simulink model "test_feng_ct_packetise"  (Simulink 7.2)
settings: Solver=ode45  StartTime=0.0  StopTime=66000  RelTol=1e-3
libraries: xbsIndex_r4 x152, xps_library x3, casper_library x3
(part 1 of 2)
settings Model: Creator=root  LastModifiedBy=root

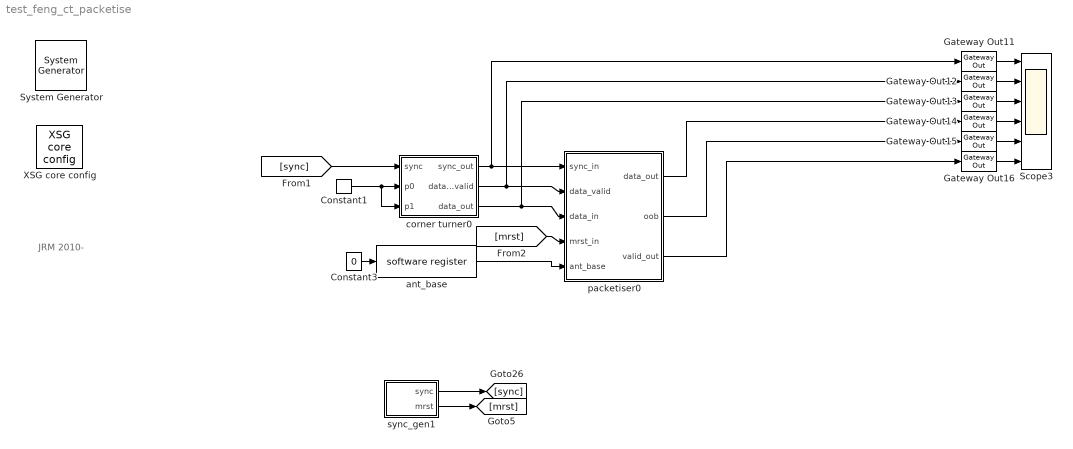
== system test_feng_ct_packetise ==
  note: JRM
      | 2010-
  " System Generator" : xbsIndex_r4/ System Generator  Tag=genX  SystemSampleTime=-1  xilinxfamily=virtex5  part=xc5vsx95t  speed=-1  package=ff1136  synthesis_tool=XST  clock_wrapper=Clock Enables  directory=./r_128w_512_11_r354/sysgen  testbench=off  simulink_period=1  sysclk_period=5  dcm_input_clock_period=100  incr_netlist=off  trim_vbits=Everywhere in SubSystem  dbl_ovrd=According to Block Masks  core_generation=According to Block Masks  run_coregen=off  deprecated_control=off  eval_field=0  block_type=sysgen
      settings: block_version=10.1.3
  Constant1 : xbsIndex_r4/Constant  arith_type=Unsigned  const=0  n_bits=16  bin_pt=0  explicit_period=off  period=1  equ=P=C  opselect=C  inp2=PCIN>>17  opr=+  inp1=P  carry=CIN  dbl_ovrd=off  block_type=constant
  Constant3 : Constant  Value=0  OutDataType=sfix(16)  OutScaling=2^0
  Gateway Out{11..16} (6 alike) : xbsIndex_r4/Gateway Out  hdl_port=off  timing_constraint=None  locs_specified=off  LOCs={}  block_type=gatewayout
      settings: infoedit="Gateway out block.  Converts Xilinx fixed point inputs into ouputs of type Simulink integer, double, or fixed point.<P><P>Hardware notes:  In hardware these blocks become top level output ports or are discarded, depending on how they are configured."  block_version=10.1.3
  Scope3 : Scope  NumInputPorts=6
      settings: YMin=-1~-1~-1~-1~-1~-1  YMax=1~1~1~1~1~1
  XSG core config : xps_library/XSG core config  Tag=xps:xsg  SystemSampleTime=-1  hw_sys=ROACH:sx95t  ibob_linux=off  clk_src=adc0_clk  iBOB_clk_src=sys_clk  BEE2_ctrl_clk_src=sys_clk  BEE2_usr_clk_src=sys_clk  ROACH_clk_src=adc0_clk  CORR_clk_src=sys_clk  gpio_clk_io_group=iBOB:sma  gpio_clk_bit_index=0  clk_rate=800/4  sample_period=1  synthesis_tool=XST  mpc_type=powerpc440_ext
  ant_base : xps_library/software register  Tag=xps:sw_reg  SystemSampleTime=-1  io_dir=From Processor  arith_type=Unsigned  bitwidth=32  bin_pt=0  sample_period=1  gw_name=test_feng_ct_packetise_ant_base_user_data_out
  corner turner0 : Subsystem  mask{num_channels_bits=6, num_spectra_bits=7, which_qdr=qdr0}
      mask prompts: num_channels_bits "Number of freq channels (total 2^?):"; num_spectra_bits "Number of spectra per XAUI packet (2^?):"; which_qdr "QDR to use:"
      mask init:
      | set_param([gcb, '/qdr_ct'], 'which_qdr', which_qdr);
      mask StyleString: edit,edit,popup(qdr0|qdr1)
  packetiser0 : Subsystem  mask{num_spectra_bits=7, ant_bits=1, ant=0}
      mask prompts: num_spectra_bits "Payload length in 64bit words (2^n):"; ant_bits "Number of dual-pol antennas per board (2^n)"; ant "This is antenna number"
      mask help: Package 32 bit data into 64 bits and identify data as coming from antenna 0 or 1
  sync_gen1 : Subsystem
  wires:
  corner turner0/3(data_out) -> Gateway Out13/1, packetiser0/3(data_in)
  corner turner0/2(data_valid) -> Gateway Out12/1, packetiser0/2(data_valid)
  Constant3/1 -> ant_base/1
  ant_base/1 -> packetiser0/5(ant_base)
  Constant1/1 -> corner turner0/3(p1), corner turner0/2(p0)
  [sync] -> corner turner0/1(sync)
  Gateway Out11/1 -> Scope3/1
  Gateway Out12/1 -> Scope3/2
  Gateway Out13/1 -> Scope3/3
  Gateway Out14/1 -> Scope3/4
  Gateway Out15/1 -> Scope3/5
  Gateway Out16/1 -> Scope3/6
  packetiser0/1(data_out) -> Gateway Out14/1
  packetiser0/2(oob) -> Gateway Out15/1
  packetiser0/3(valid_out) -> Gateway Out16/1
  corner turner0/1(sync_out) -> Gateway Out11/1, packetiser0/1(sync_in)
  [mrst] -> packetiser0/4(mrst_in)
  sync_gen1/2(mrst) -> [mrst]
  sync_gen1/1(sync) -> [sync]

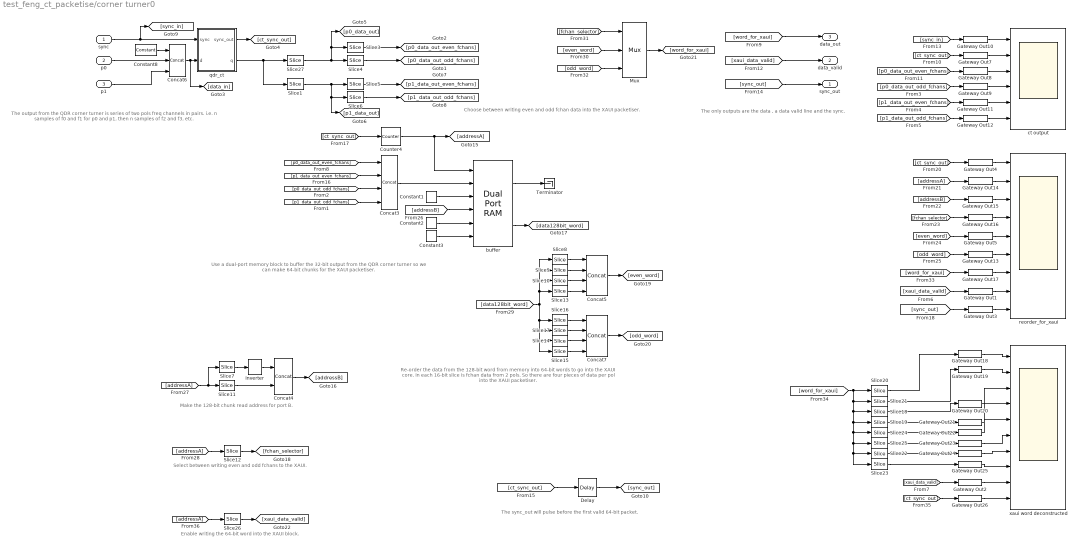
== system test_feng_ct_packetise/corner turner0 ==
  note: Make the 128-bit chunk read address for port B.
  note: Select between writing even and odd fchans to the XAUI.
  note: Re-order the data from the 128-bit word from memory
      | into 64-bit words to go into the XAUI core.
      | In each 16-bit slice is fchan data from 2 pols. So there
      | are four pieces of data per pol into the XAUI packetiser.
  note: Enable writing the 64-bit word into the XAUI block.
  note: The output from the QDR corner turner is series of two pols freq channels in pairs.
      | i.e. n samples of f0 and f1 for p0 and p1, then n samples of f2 and f3, etc.
  note: Use a dual-port memory block to buffer the 32-bit output from the
      | QDR corner turner so we can make 64-bit chunks for the XAUI packetiser.
  note: Choose between writing even and odd fchan data into
      | the XAUI packetiser.
  note: The only outputs are the data , a data valid line and the sync.
  note: The sync_out will pulse before the first valid 64-bit packet.
  sync : Inport  OutDataType=sfix(16)  OutScaling=2^0
  p0 : Inport  Port=2  OutDataType=sfix(16)  OutScaling=2^0
  p1 : Inport  Port=3  OutDataType=sfix(16)  OutScaling=2^0
  Concat3 : xbsIndex_r4/Concat  num_inputs=4  dbl_ovrd=off  block_type=concat
      settings: block_version=10.1.3
  Concat4 : xbsIndex_r4/Concat  num_inputs=2  dbl_ovrd=off  block_type=concat
      settings: block_version=10.1.3
  Concat5 : xbsIndex_r4/Concat  num_inputs=4  dbl_ovrd=off  block_type=concat
      settings: block_version=10.1.3
  Concat6 : xbsIndex_r4/Concat  num_inputs=3  dbl_ovrd=off  block_type=concat
      settings: block_version=10.1.3
  Concat7 : xbsIndex_r4/Concat  num_inputs=4  dbl_ovrd=off  block_type=concat
      settings: block_version=10.1.3
  Constant1 : xbsIndex_r4/Constant  arith_type=Boolean  const=1  n_bits=4  bin_pt=0  explicit_period=off  period=1  equ=P=C  opselect=C  inp2=PCIN>>17  opr=+  inp1=P  carry=CIN  dbl_ovrd=off  block_type=constant
  Constant2 : xbsIndex_r4/Constant  arith_type=Unsigned  const=0  n_bits=128  bin_pt=0  explicit_period=off  period=1  equ=P=C  opselect=C  inp2=PCIN>>17  opr=+  inp1=P  carry=CIN  dbl_ovrd=off  block_type=constant
  Constant3 : xbsIndex_r4/Constant  arith_type=Boolean  const=0  n_bits=64  bin_pt=0  explicit_period=off  period=1  equ=P=C  opselect=C  inp2=PCIN>>17  opr=+  inp1=P  carry=CIN  dbl_ovrd=off  block_type=constant
  Constant8 : xbsIndex_r4/Constant  arith_type=Unsigned  const=0  n_bits=4  bin_pt=0  explicit_period=off  period=1  equ=P=C  opselect=C  inp2=PCIN>>17  opr=+  inp1=P  carry=CIN  dbl_ovrd=off  block_type=constant
  Counter4 : xbsIndex_r4/Counter  cnt_type=Free Running  cnt_to=Inf  operation=Up  start_count=0  cnt_by_val=1  arith_type=Unsigned  n_bits=num_spectra_bits + 1  bin_pt=0  load_pin=off  rst=on  en=off  explicit_period=on  period=1  dbl_ovrd=off  use_behavioral_HDL=off  implementation=Fabric  block_type=counter
      settings: block_version=11.4
  Delay : xbsIndex_r4/Delay  en=off  latency=2 ^ num_spectra_bits +1  dbl_ovrd=off  reg_retiming=off  block_type=delay
      settings: block_version=11.4
  Gateway Out{1..5,7..26} (25 alike) : xbsIndex_r4/Gateway Out  hdl_port=on  timing_constraint=None  locs_specified=off  LOCs={}  block_type=gatewayout
      settings: infoedit="Gateway out block.  Converts Xilinx fixed point inputs into ouputs of type Simulink integer, double, or fixed point.<br><br>Hardware notes:  In hardware these blocks become top level output ports or are discarded, depending on how they are configured."  block_version=11.4
  Inverter : xbsIndex_r4/Inverter  en=off  latency=0  dbl_ovrd=off  block_type=inv
      settings: block_version=11.4
  Mux : xbsIndex_r4/Mux  inputs=2  en=off  latency=0  precision=Full  arith_type=Unsigned  n_bits=16  bin_pt=14  quantization=Truncate  overflow=Wrap  dbl_ovrd=off  block_type=mux
      settings: block_version=11.4
  Slice1 : xbsIndex_r4/Slice  nbits=16  boolean_output=off  mode=Lower Bit Location + Width  bit1=0  base1=MSB of Input  bit0=0  base0=LSB of Input  dbl_ovrd=off  block_type=slice
      settings: block_version=10.1.3
  Slice10 : xbsIndex_r4/Slice  nbits=16  boolean_output=off  mode=Upper Bit Location + Width  bit1=-64  base1=MSB of Input  bit0=1  base0=LSB of Input  dbl_ovrd=off  block_type=slice
      settings: block_version=10.1.3
  Slice11 : xbsIndex_r4/Slice  nbits=num_spectra_bits - 2  boolean_output=off  mode=Lower Bit Location + Width  bit1=0  base1=MSB of Input  bit0=1  base0=LSB of Input  dbl_ovrd=off  block_type=slice
      settings: block_version=10.1.3
  Slice12 : xbsIndex_r4/Slice  nbits=1  boolean_output=on  mode=Upper Bit Location + Width  bit1=-1  base1=MSB of Input  bit0=1  base0=LSB of Input  dbl_ovrd=off  block_type=slice
      settings: block_version=10.1.3
  Slice13 : xbsIndex_r4/Slice  nbits=16  boolean_output=off  mode=Upper Bit Location + Width  bit1=-96  base1=MSB of Input  bit0=1  base0=LSB of Input  dbl_ovrd=off  block_type=slice
      settings: block_version=10.1.3
  Slice14 : xbsIndex_r4/Slice  nbits=16  boolean_output=off  mode=Upper Bit Location + Width  bit1=-80  base1=MSB of Input  bit0=1  base0=LSB of Input  dbl_ovrd=off  block_type=slice
      settings: block_version=10.1.3
  Slice15 : xbsIndex_r4/Slice  nbits=16  boolean_output=off  mode=Upper Bit Location + Width  bit1=-112  base1=MSB of Input  bit0=1  base0=LSB of Input  dbl_ovrd=off  block_type=slice
      settings: block_version=10.1.3
  Slice16 : xbsIndex_r4/Slice  nbits=16  boolean_output=off  mode=Upper Bit Location + Width  bit1=-16  base1=MSB of Input  bit0=1  base0=LSB of Input  dbl_ovrd=off  block_type=slice
      settings: block_version=10.1.3
  Slice17 : xbsIndex_r4/Slice  nbits=16  boolean_output=off  mode=Upper Bit Location + Width  bit1=-48  base1=MSB of Input  bit0=1  base0=LSB of Input  dbl_ovrd=off  block_type=slice
      settings: block_version=10.1.3
  Slice18 : xbsIndex_r4/Slice  nbits=8  boolean_output=off  mode=Lower Bit Location + Width  bit1=-64  base1=MSB of Input  bit0=40  base0=LSB of Input  dbl_ovrd=off  block_type=slice
      settings: block_version=10.1.3
  Slice19 : xbsIndex_r4/Slice  nbits=8  boolean_output=off  mode=Lower Bit Location + Width  bit1=-96  base1=MSB of Input  bit0=32  base0=LSB of Input  dbl_ovrd=off  block_type=slice
      settings: block_version=10.1.3
  Slice20 : xbsIndex_r4/Slice  nbits=8  boolean_output=off  mode=Lower Bit Location + Width  bit1=0  base1=MSB of Input  bit0=56  base0=LSB of Input  dbl_ovrd=off  block_type=slice
      settings: block_version=10.1.3
  Slice21 : xbsIndex_r4/Slice  nbits=8  boolean_output=off  mode=Lower Bit Location + Width  bit1=-8  base1=MSB of Input  bit0=48  base0=LSB of Input  dbl_ovrd=off  block_type=slice
      settings: block_version=10.1.3
  Slice22 : xbsIndex_r4/Slice  nbits=8  boolean_output=off  mode=Lower Bit Location + Width  bit1=-64  base1=MSB of Input  bit0=0  base0=LSB of Input  dbl_ovrd=off  block_type=slice
      settings: block_version=10.1.3
  Slice23 : xbsIndex_r4/Slice  nbits=8  boolean_output=off  mode=Lower Bit Location + Width  bit1=-96  base1=MSB of Input  bit0=0  base0=LSB of Input  dbl_ovrd=off  block_type=slice
      settings: block_version=10.1.3
  Slice24 : xbsIndex_r4/Slice  nbits=8  boolean_output=off  mode=Lower Bit Location + Width  bit1=0  base1=MSB of Input  bit0=24  base0=LSB of Input  dbl_ovrd=off  block_type=slice
      settings: block_version=10.1.3
  Slice25 : xbsIndex_r4/Slice  nbits=8  boolean_output=off  mode=Lower Bit Location + Width  bit1=8  base1=MSB of Input  bit0=16  base0=LSB of Input  dbl_ovrd=off  block_type=slice
      settings: block_version=10.1.3
  Slice26 : xbsIndex_r4/Slice  nbits=1  boolean_output=on  mode=Lower Bit Location + Width  bit1=-1  base1=MSB of Input  bit0=0  base0=LSB of Input  dbl_ovrd=off  block_type=slice
      settings: block_version=10.1.3
  Slice27 : xbsIndex_r4/Slice  nbits=16  boolean_output=off  mode=Lower Bit Location + Width  bit1=0  base1=MSB of Input  bit0=16  base0=LSB of Input  dbl_ovrd=off  block_type=slice
      settings: block_version=10.1.3
  Slice3 : xbsIndex_r4/Slice  nbits=8  boolean_output=off  mode=Lower Bit Location + Width  bit1=0  base1=MSB of Input  bit0=8  base0=LSB of Input  dbl_ovrd=off  block_type=slice
      settings: block_version=10.1.3
  Slice4 : xbsIndex_r4/Slice  nbits=8  boolean_output=off  mode=Lower Bit Location + Width  bit1=0  base1=MSB of Input  bit0=0  base0=LSB of Input  dbl_ovrd=off  block_type=slice
      settings: block_version=10.1.3
  Slice5 : xbsIndex_r4/Slice  nbits=8  boolean_output=off  mode=Lower Bit Location + Width  bit1=0  base1=MSB of Input  bit0=8  base0=LSB of Input  dbl_ovrd=off  block_type=slice
      settings: block_version=10.1.3
  Slice6 : xbsIndex_r4/Slice  nbits=8  boolean_output=off  mode=Lower Bit Location + Width  bit1=0  base1=MSB of Input  bit0=0  base0=LSB of Input  dbl_ovrd=off  block_type=slice
      settings: block_version=10.1.3
  Slice7 : xbsIndex_r4/Slice  nbits=1  boolean_output=off  mode=Upper Bit Location + Width  bit1=0  base1=MSB of Input  bit0=1  base0=LSB of Input  dbl_ovrd=off  block_type=slice
      settings: block_version=10.1.3
  Slice8 : xbsIndex_r4/Slice  nbits=16  boolean_output=off  mode=Upper Bit Location + Width  bit1=0  base1=MSB of Input  bit0=1  base0=LSB of Input  dbl_ovrd=off  block_type=slice
      settings: block_version=10.1.3
  Slice9 : xbsIndex_r4/Slice  nbits=16  boolean_output=off  mode=Upper Bit Location + Width  bit1=-32  base1=MSB of Input  bit0=1  base0=LSB of Input  dbl_ovrd=off  block_type=slice
      settings: block_version=10.1.3
  Terminator : Terminator
  buffer : xbsIndex_r4/Dual Port RAM  depth=(2 ^ num_spectra_bits) * 2  initVector=sin(pi*(0:15)/16)  distributed_mem=Block RAM  init_a=0  init_b=0  rst_a=off  rst_b=off  en_a=off  en_b=off  latency=1  write_mode_A=Read Before Write  write_mode_B=Read Before Write  dbl_ovrd=off  optimize=Area  use_rpm=on  block_type=dpram
      settings: block_version=11.4
  ct output : Scope  NumInputPorts=6
      settings: YMin=-5~-5~-10~-5~-5~-5  YMax=5~5~300~5~5~5  MaxDataPoints=100000
  qdr_ct : Subsystem  AncestorBlock=casper_library/Reorder/qdr_transpose  mask{idepth=num_channels_bits - 1, odepth=num_spectra_bits, which_qdr=qdr0}
      mask prompts: idepth "Input blocksize (2^n)"; odepth "Output blocksize (2^n)"; which_qdr "QDR to use:"
      mask init:
      | new_map = tostring([[0:2^odepth-1]*2 [0:2^odepth-1]*2 + 1]);
      | set_param([gcb, '/reorder'], 'map', new_map);
      | set_param([gcb, '/qdr'], 'which_qdr', which_qdr);
      mask StyleString: edit,edit,popup(qdr0|qdr1)
  reorder_for_xaui : Scope  NumInputPorts=9
      settings: YMin=-1~-5~-10~-0.1~-5~-5~-5~-0.1~-5  YMax=2~5~300~1.1~5~5~5~1.1~5  SaveName=ScopeData3  MaxDataPoints=100000
  xaui word deconstructed : Scope  NumInputPorts=10
      settings: YMin=-1~-5~-10~-0.1~-5~-5~-5~-5~-0.1~-5  YMax=2~5~300~1.1~5~5~5~5~1.1~5  SaveName=ScopeData4  MaxDataPoints=100000
  sync_out : Outport  OutDataType=sfix(16)  OutScaling=2^0
  data_valid : Outport  Port=2  OutDataType=sfix(16)  OutScaling=2^0
  data_out : Outport  Port=3  OutDataType=sfix(16)  OutScaling=2^0
  wires:
  p0/1 -> Concat6/2
  p1/1 -> Concat6/3
  Constant8/1 -> Concat6/1
  sync/1 -> qdr_ct/1(sync), [sync_in]
  Concat6/1 -> qdr_ct/2(d), [data_in]
  qdr_ct/1(sync_out) -> [ct_sync_out]
  qdr_ct/2(q) -> Slice27/1, Slice1/1
  Slice27/1 -> Slice4/1, [p0_data_out], Slice3/1
  Slice1/1 -> Slice5/1, [p1_data_out], Slice6/1
  Slice3/1 -> [p0_data_out_even_fchans]
  Slice4/1 -> [p0_data_out_odd_fchans]
  Slice5/1 -> [p1_data_out_even_fchans]
  Slice6/1 -> [p1_data_out_odd_fchans]
  [ct_sync_out] -> Gateway Out7/1
  [p0_data_out_even_fchans] -> Gateway Out8/1
  [p0_data_out_odd_fchans] -> Gateway Out9/1
  [sync_in] -> Gateway Out10/1
  [p1_data_out_even_fchans] -> Gateway Out11/1
  [p1_data_out_odd_fchans] -> Gateway Out12/1
  Gateway Out7/1 -> ct output/2
  Gateway Out10/1 -> ct output/1
  Gateway Out8/1 -> ct output/3
  Gateway Out9/1 -> ct output/4
  Gateway Out11/1 -> ct output/5
  Gateway Out12/1 -> ct output/6
  [p0_data_out_even_fchans] -> Concat3/1
  [p1_data_out_even_fchans] -> Concat3/2
  Concat3/1 -> buffer/2
  [ct_sync_out] -> Counter4/1
  Constant1/1 -> buffer/3
  Constant2/1 -> buffer/5
  Constant3/1 -> buffer/6
  [p0_data_out_odd_fchans] -> Concat3/3
  [p1_data_out_odd_fchans] -> Concat3/4
  buffer/1 -> Terminator/1
  Gateway Out4/1 -> reorder_for_xaui/1
  Gateway Out14/1 -> reorder_for_xaui/2
  Gateway Out15/1 -> reorder_for_xaui/3
  Gateway Out16/1 -> reorder_for_xaui/4
  Gateway Out5/1 -> reorder_for_xaui/5
  Gateway Out13/1 -> reorder_for_xaui/6
  [ct_sync_out] -> Gateway Out4/1
  [addressA] -> Gateway Out14/1
  [addressB] -> Gateway Out15/1
  [fchan_selector] -> Gateway Out16/1
  [even_word] -> Gateway Out5/1
  [odd_word] -> Gateway Out13/1
  Mux/1 -> [word_for_xaui]
  [addressB] -> buffer/4
  [addressA] -> Slice11/1, Slice7/1
  Slice11/1 -> Concat4/2
  Slice7/1 -> Inverter/1
  Inverter/1 -> Concat4/1
  Concat4/1 -> [addressB]
  [addressA] -> Slice12/1
  Slice12/1 -> [fchan_selector]
  buffer/2 -> [data128bit_word]
  Slice8/1 -> Concat5/1
  Slice9/1 -> Concat5/2
  Slice10/1 -> Concat5/3
  Slice13/1 -> Concat5/4
  [data128bit_word] -> Slice8/1, Slice9/1, Slice10/1, Slice13/1, Slice16/1, Slice17/1, Slice14/1, Slice15/1
  Slice16/1 -> Concat7/1
  Slice17/1 -> Concat7/2
  Slice14/1 -> Concat7/3
  Slice15/1 -> Concat7/4
  Concat5/1 -> [even_word]
  Concat7/1 -> [odd_word]
  [even_word] -> Mux/2
  [fchan_selector] -> Mux/1
  [odd_word] -> Mux/3
  [word_for_xaui] -> Gateway Out17/1
  Gateway Out17/1 -> reorder_for_xaui/7
  [word_for_xaui] -> Slice20/1, Slice21/1, Slice18/1, Slice19/1, Slice24/1, Slice25/1, Slice22/1, Slice23/1
  Slice20/1 -> Gateway Out18/1
  Slice21/1 -> Gateway Out19/1
  Slice18/1 -> Gateway Out20/1
  Slice19/1 -> Gateway Out21/1
  Slice24/1 -> Gateway Out22/1
  Slice25/1 -> Gateway Out23/1
  Slice22/1 -> Gateway Out24/1
  Slice23/1 -> Gateway Out25/1
  Gateway Out18/1 -> xaui word deconstructed/1
  Gateway Out19/1 -> xaui word deconstructed/2
  Gateway Out20/1 -> xaui word deconstructed/3
  Gateway Out21/1 -> xaui word deconstructed/4
  Gateway Out22/1 -> xaui word deconstructed/5
  Gateway Out23/1 -> xaui word deconstructed/6
  Gateway Out24/1 -> xaui word deconstructed/7
  Gateway Out25/1 -> xaui word deconstructed/8
  [ct_sync_out] -> Gateway Out26/1
  [addressA] -> Slice26/1
  Slice26/1 -> [xaui_data_valid]
  Counter4/1 -> buffer/1, [addressA]
  [xaui_data_valid] -> Gateway Out1/1
  Gateway Out1/1 -> reorder_for_xaui/8
  [xaui_data_valid] -> Gateway Out2/1
  Gateway Out2/1 -> xaui word deconstructed/9
  Gateway Out26/1 -> xaui word deconstructed/10
  [word_for_xaui] -> data_out/1
  [xaui_data_valid] -> data_valid/1
  [sync_out] -> sync_out/1
  [ct_sync_out] -> Delay/1
  Delay/1 -> [sync_out]
  [sync_out] -> Gateway Out3/1
  Gateway Out3/1 -> reorder_for_xaui/9

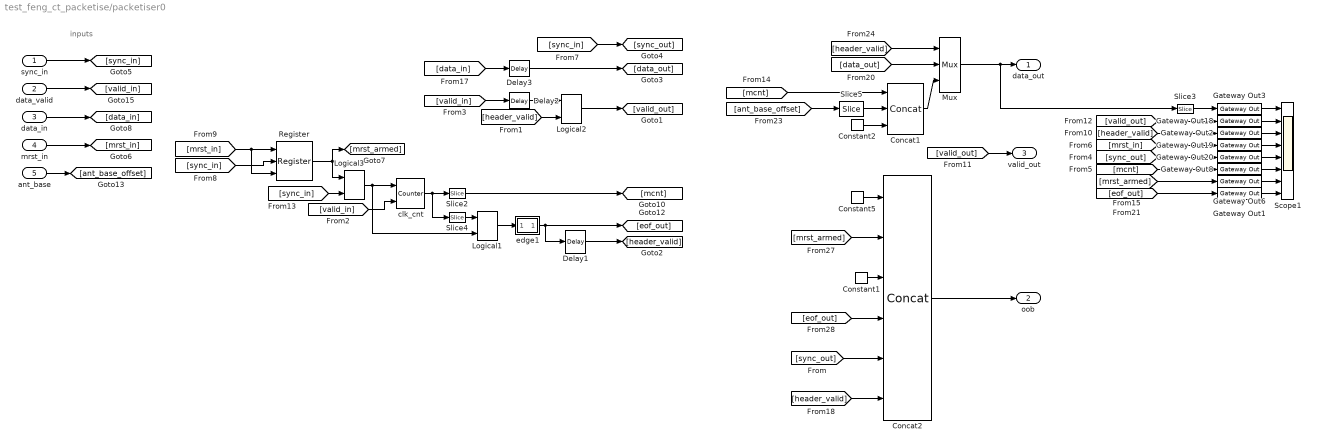
== system test_feng_ct_packetise/packetiser0 ==
  note: inputs
  sync_in : Inport  OutDataType=sfix(16)  OutScaling=2^0
  data_valid : Inport  Port=2  OutDataType=sfix(16)  OutScaling=2^0
  data_in : Inport  Port=3  OutDataType=sfix(16)  OutScaling=2^0
  mrst_in : Inport  Port=4  OutDataType=sfix(16)  OutScaling=2^0
  ant_base : Inport  Port=5  OutDataType=sfix(16)  OutScaling=2^0
  Concat1 : xbsIndex_r4/Concat  num_inputs=3  dbl_ovrd=off  block_type=concat
      settings: block_version=10.1.3
  Concat2 : xbsIndex_r4/Concat  num_inputs=6  dbl_ovrd=off  block_type=concat
      settings: block_version=10.1.3
  Constant1 : xbsIndex_r4/Constant  arith_type=Unsigned  const=0  n_bits=1  bin_pt=0  explicit_period=off  period=1  equ=P=C  opselect=C  inp2=PCIN>>17  opr=+  inp1=P  carry=CIN  dbl_ovrd=off  block_type=constant
  Constant2 : xbsIndex_r4/Constant  arith_type=Unsigned  const=ant  n_bits=ant_bits  bin_pt=0  explicit_period=off  period=1  equ=P=C  opselect=C  inp2=PCIN>>17  opr=+  inp1=P  carry=CIN  dbl_ovrd=off  block_type=constant
  Constant5 : xbsIndex_r4/Constant  arith_type=Unsigned  const=0  n_bits=3  bin_pt=0  explicit_period=off  period=1  equ=P=C  opselect=C  inp2=PCIN>>17  opr=+  inp1=P  carry=CIN  dbl_ovrd=off  block_type=constant
  Delay1 : xbsIndex_r4/Delay  en=off  latency=1  dbl_ovrd=off  reg_retiming=on  block_type=delay
      settings: xl_area=[0, 0, 0, 0, 0, 0, 0]
  Delay2 : xbsIndex_r4/Delay  en=off  latency=1  dbl_ovrd=off  reg_retiming=on  block_type=delay
      settings: xl_area=[0, 0, 0, 0, 0, 0, 0]
  Delay3 : xbsIndex_r4/Delay  en=off  latency=1  dbl_ovrd=off  reg_retiming=on  block_type=delay
      settings: xl_area=[0, 0, 0, 0, 0, 0, 0]
  Gateway Out{1..3,6,8,18..20} (8 alike) : xbsIndex_r4/Gateway Out  hdl_port=on  timing_constraint=None  locs_specified=off  LOCs={}  block_type=gatewayout
      settings: infoedit="Gateway out block.  Converts Xilinx fixed point inputs into ouputs of type Simulink integer, double, or fixed point.<P><P>Hardware notes:  In hardware these blocks become top level output ports or are discarded, depending on how they are configured."  xl_area=[0, 0, 0, 0, 0, 0, 0]  block_version=10.1.3
  Logical1 : xbsIndex_r4/Logical  logical_function=OR  inputs=2  en=off  latency=0  precision=Full  arith_type=Unsigned  n_bits=1  bin_pt=0  align_bp=on  dbl_ovrd=off  block_type=logical
      settings: xl_area=[0, 0, 0, 0, 0, 0, 0]
  Logical2 : xbsIndex_r4/Logical  logical_function=OR  inputs=2  en=off  latency=0  precision=Full  arith_type=Unsigned  n_bits=1  bin_pt=0  align_bp=on  dbl_ovrd=off  block_type=logical
      settings: xl_area=[0, 0, 0, 0, 0, 0, 0]
  Logical3 : xbsIndex_r4/Logical  logical_function=AND  inputs=2  en=off  latency=0  precision=Full  arith_type=Unsigned  n_bits=1  bin_pt=0  align_bp=on  dbl_ovrd=off  block_type=logical
      settings: xl_area=[0, 0, 0, 0, 0, 0, 0]
  Mux : xbsIndex_r4/Mux  inputs=2  en=off  latency=0  precision=Full  arith_type="Signed  (2's comp)"  n_bits=8  bin_pt=2  quantization=Truncate  overflow=Wrap  dbl_ovrd=off  block_type=mux
      settings: xl_area=[0, 0, 0, 0, 0, 0, 0]
  Register : xbsIndex_r4/Register  init=0  rst=on  en=on  dbl_ovrd=off  block_type=register
      settings: xl_area=[0, 0, 0, 0, 0, 0, 0]
  Scope1 : Scope  NumInputPorts=8
      settings: YMin=0~0~0~-1~0~100~-1~0  YMax=7.5e+07~1~1~1~1~1000~1~1  SaveName=ScopeData5
  Slice2 : xbsIndex_r4/Slice  nbits=48  boolean_output=off  mode=Upper Bit Location + Width  bit1=0  base1=MSB of Input  bit0=0  base0=LSB of Input  dbl_ovrd=off  block_type=slice
      settings: infoedit="Extracts a given range of bits from each input sample and presents it at the output.  The output type is ordinarily unsigned with binary point at zero, but can be Boolean when the slice is one bit wide.<P><P>Hardware notes: In hardware this block costs nothing."  block_version=10.1.3
  Slice3 : xbsIndex_r4/Slice  nbits=32  boolean_output=off  mode=Lower Bit Location + Width  bit1=0  base1=MSB of Input  bit0=0  base0=LSB of Input  dbl_ovrd=off  block_type=slice
      settings: infoedit="Extracts a given range of bits from each input sample and presents it at the output.  The output type is ordinarily unsigned with binary point at zero, but can be Boolean when the slice is one bit wide.<P><P>Hardware notes: In hardware this block costs nothing."  block_version=10.1.3
  Slice4 : xbsIndex_r4/Slice  nbits=1  boolean_output=on  mode=Lower Bit Location + Width  bit1=0  base1=MSB of Input  bit0=num_spectra_bits - 2  base0=LSB of Input  dbl_ovrd=off  block_type=slice
      settings: block_version=10.1.3
  Slice5 : xbsIndex_r4/Slice  nbits=16-ant_bits  boolean_output=off  mode=Lower Bit Location + Width  bit1=0  base1=LSB of Input  bit0=0  base0=LSB of Input  dbl_ovrd=off  block_type=slice
      settings: block_version=10.1.3
  clk_cnt : xbsIndex_r4/Counter  cnt_type=Free Running  cnt_to=Inf  operation=Up  start_count=0  cnt_by_val=1  arith_type=Unsigned  n_bits=48 + (num_spectra_bits-2)  bin_pt=0  load_pin=off  rst=on  en=on  explicit_period=off  period=1  dbl_ovrd=off  use_behavioral_HDL=off  implementation=Fabric  use_rpm=on  block_type=counter
      settings: xl_area=[0, 0, 0, 0, 0, 0, 0]
  edge1 : Subsystem
      mask Type: edge
      mask Description: Outputs true if a boolean input signal is not equal to its value last clock.
      mask Help: eval('xlWeb([getenv(''MLIB_ROOT''), ''\casper_library\doc\edge_usage.html''])')
  data_out : Outport  OutDataType=sfix(16)  OutScaling=2^0
  oob : Outport  Port=2  OutDataType=sfix(16)  OutScaling=2^0
  valid_out : Outport  Port=3  OutDataType=sfix(16)  OutScaling=2^0
  wires:
  Delay3/1 -> [data_out]
  [data_in] -> Delay3/1
  Delay2/1 -> Logical2/1
  Logical3/1 -> Logical1/2, clk_cnt/1
  Register/1 -> [mrst_armed], Logical3/1
  [sync_in] -> Logical3/2
  [valid_out] -> valid_out/1
  Logical2/1 -> [valid_out]
  Slice3/1 -> Gateway Out3/1
  Gateway Out3/1 -> Scope1/1
  [header_valid] -> Logical2/2
  Delay1/1 -> [header_valid]
  [valid_in] -> Delay2/1
  [valid_in] -> clk_cnt/2
  Mux/1 -> Slice3/1, data_out/1
  [header_valid] -> Concat2/6
  Constant2/1 -> Concat1/3
  Constant5/1 -> Concat2/1
  Constant1/1 -> Concat2/3
  [mrst_armed] -> Concat2/2
  [sync_out] -> Concat2/5
  [eof_out] -> Concat2/4
  Concat2/1 -> oob/1
  [header_valid] -> Mux/1
  [data_out] -> Mux/2
  [sync_in] -> [sync_out]
  edge1/1(out) -> Delay1/1, [eof_out]
  Logical1/1 -> edge1/1(in)
  Slice4/1 -> Logical1/1
  Slice2/1 -> [mcnt]
  clk_cnt/1 -> Slice4/1, Slice2/1
  [sync_in] -> Register/2
  [mrst_in] -> Register/3, Register/1
  [ant_base_offset] -> Slice5/1
  [mcnt] -> Concat1/1
  Concat1/1 -> Mux/3
  Slice5/1 -> Concat1/2
  data_valid/1 -> [valid_in]
  ant_base/1 -> [ant_base_offset]
  data_in/1 -> [data_in]
  mrst_in/1 -> [mrst_in]
  sync_in/1 -> [sync_in]
  Gateway Out18/1 -> Scope1/2
  Gateway Out2/1 -> Scope1/3
  Gateway Out19/1 -> Scope1/4
  Gateway Out20/1 -> Scope1/5
  [header_valid] -> Gateway Out2/1
  [mrst_in] -> Gateway Out19/1
  [sync_out] -> Gateway Out20/1
  Gateway Out8/1 -> Scope1/6
  [mcnt] -> Gateway Out8/1
  Gateway Out6/1 -> Scope1/7
  Gateway Out1/1 -> Scope1/8
  [eof_out] -> Gateway Out1/1
  [valid_out] -> Gateway Out18/1
  [mrst_armed] -> Gateway Out6/1

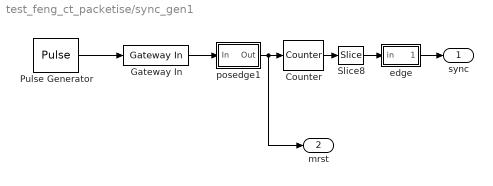
== system test_feng_ct_packetise/sync_gen1 ==
  Counter : xbsIndex_r4/Counter  cnt_type=Free Running  cnt_to=Inf  operation=Up  start_count=0  cnt_by_val=1  arith_type=Unsigned  n_bits=15  bin_pt=0  load_pin=off  rst=on  en=off  explicit_period=off  period=1  dbl_ovrd=off  use_behavioral_HDL=off  implementation=Fabric  use_rpm=on  block_type=counter
      settings: xl_area=[0, 0, 0, 0, 0, 0, 0]
  Gateway In : xbsIndex_r4/Gateway In  arith_type=Boolean  n_bits=16  bin_pt=14  quantization="Round  (unbiased: +/- Inf)"  overflow=Saturate  period=1  dbl_ovrd=off  timing_constraint=None  locs_specified=off  LOCs={}  hdl_port=on  block_type=gatewayin
      settings: infoedit="Gateway in block.  Converts inputs of type Simulink integer, double and fixed point to  Xilinx fixed point type.<br><br>Hardware notes:  In hardware these blocks become top level input ports."  block_version=11.4
  Pulse Generator : DiscretePulseGenerator  Period=2^17  PhaseDelay=1
  Slice8 : xbsIndex_r4/Slice  nbits=1  boolean_output=on  mode=Upper Bit Location + Width  bit1=0  base1=MSB of Input  bit0=19  base0=LSB of Input  dbl_ovrd=off  block_type=slice
      settings: infoedit="Extracts a given range of bits from each input sample and presents it at the output.  The output type is ordinarily unsigned with binary point at zero, but can be Boolean when the slice is one bit wide.<P><P>Hardware notes: In hardware this block costs nothing."  block_version=10.1.3
  edge : Subsystem
  posedge1 : Subsystem  Tag=Rising Edge Detector
  sync : Outport  OutDataType=sfix(16)  OutScaling=2^0
  mrst : Outport  Port=2  OutDataType=sfix(16)  OutScaling=2^0
  wires:
  Counter/1 -> Slice8/1
  posedge1/1(Out) -> Counter/1, mrst/1
  Slice8/1 -> edge/1(in)
  edge/1(out) -> sync/1
  Gateway In/1 -> posedge1/1(In)
  Pulse Generator/1 -> Gateway In/1
